simulink subsystem "BatteryHighGroupedRefSub"  (R2022a)
settings: Solver=VariableStepAuto  StartTime=0.0  StopTime=10.0  RelTol=1e-3
undefined symbols (not defined in the file): batteryHV
libraries: fl_lib x8, nesl_utility x7, batteryModule_lib x1
settings Model: Creator=jjha  LastModifiedBy=jjha
settings SolverCC: AlgebraicLoopSolver=TrustRegion
settings DebuggingCC: UnconnectedInputMsg=warning  UnconnectedOutputMsg=warning  UnconnectedLineMsg=warning
settings RTWCC: DLArmComputeVersion=19.05

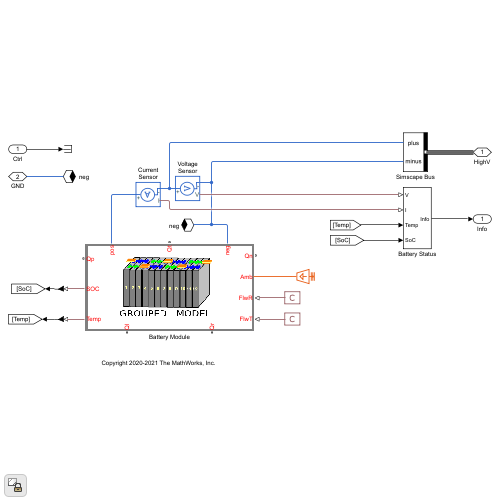
[thumbnail: Simulink's stored preview of the top-level diagram]
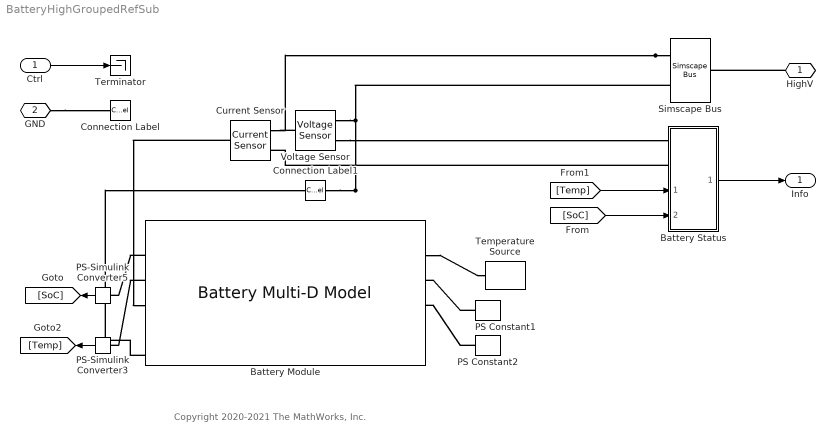
== system BatteryHighGroupedRefSub ==
  note: Copyright 2020-2021 The MathWorks, Inc.
  Ctrl : Inport
  Battery Module : batteryModule_lib/Battery Multi-D Model  modelComplexity=batteryModule.batteryAbstractionLevel.grouped  LUTpointsTemp=batteryHV.batteryTemp_LUT K  cellAH=batteryHV.batteryCapacity_LUT A*hr  LUTpointsSOC=batteryHV.batterySOC_LUT  V0_mat=batteryHV.batteryEm_LUT V  prm_dir=ee.enum.battery.prm_dir.noCurrentDirectionality  R0_mat=batteryHV.batteryR0_LUT Ohm  R0_dis_mat=[.03, .015, .002; .04, .017, .008; .039, .012, .006; .027, .013, .021] Ohm  R0_ch_mat=[.03, .015, .002; .04, .017, .008; .039, .012, .006; .027, .013, .021] Ohm  prm_leak=ee.enum.battery.prm_leak.disabled  Rleak_vec=[8000, 7000, 6000] Ohm  extrapolation_option=simscape.enum.extrapolation.nearest  prm_dyn=ee.enum.battery.prm_dyn.rc1  R1_mat=batteryHV.batteryR1_LUT Ohm  tau1_mat=batteryHV.batteryTau1_LUT s  R2_mat=[.014, .382, .407; .028, .006, .007; .014, .007, .006; .333, .956, .912] Ohm  tau2_mat=[1, 44, 5644; 11, 24, 506; 2, 14, 330; 3310, 13419, 30216] s  R3_mat=[.014, .382, .407; .028, .006, .007; .014, .007, .006; .333, .956, .912] Ohm  tau3_mat=[1, 44, 5644; 11, 24, 506; 2, 14, 330; 3310, 13419, 30216] s  R4_mat=[.014, .382, .407; .028, .006, .007; .014, .007, .006; .333, .956, .912] Ohm  tau4_mat=[1, 44, 5644; 11, 24, 506; 2, 14, 330; 3310, 13419, 30216] s  R5_mat=[.014, .382, .407; .028, .006, .007; .014, .007, .006; .333, .956, .912] Ohm  tau5_mat=[1, 44, 5644; 11, 24, 506; 2, 14, 330; 3310, 13419, 30216] s  prm_fade=ee.enum.battery.prm_fade.equations  N0=100  dV0=0  dR0=0  dAH=0  dRleak=0  dR1=0  dR2=0  dR3=0  dR4=0  dR5=0  N0vec=[100, 200, 300]  Tfadevec=[298.15, 323.15] K  dV0vec=[0, 0, 0]  dR0vec=[0, 0, 0]  dAHvec=[0, 0, 0]  dRleakvec=[0, 0, 0]  dR1vec=[0, 0, 0]  dR2vec=[0, 0, 0]  dR3vec=[0, 0, 0]  dR4vec=[0, 0, 0]  dR5vec=[0, 0, 0]  dV0mat=[0, 0; 0, 0; 0, 0]  dR0mat=[0, 0; 0, 0; 0, 0]  dAHmat=[0, 0; 0, 0; 0, 0]  dRleakmat=[0, 0; 0, 0; 0, 0]  dR1mat=[0, 0; 0, 0; 0, 0]  dR2mat=[0, 0; 0, 0; 0, 0]  dR3mat=[0, 0; 0, 0; 0, 0]  dR4mat=[0, 0; 0, 0; 0, 0]  dR5mat=[0, 0; 0, 0; 0, 0]  cellThermalMass=batteryHV.batteryCell_mass*batteryHV.batteryCell_cp J/K  cellThermalCond=batteryHV.batteryThermal_K1 W/(m*K)  cellThermalCond_inPlane=batteryHV.batteryThermal_K2 W/(m*K)  Ns=batteryHV.batteryNs  Np=batteryHV.batteryNp  cellTypeSelection=batteryModule.batteryTypeSelection.pouch  cellHeight=batteryHV.batteryCell_H m  cellWidth=batteryHV.batteryCell_W m  cellThickness=batteryHV.batteryCell_T m  cellDiameter=0.018 m  cellCylinLine=3  moduleExternalR=batteryHV.battery_extR Ohm  moduleCellBalancing=batteryModule.batteryCellBalancing.none  passiveShuntR=50 Ohm  passiveSWclosedR=0.01 Ohm  passiveSWopenCond=1e-8 1/Ohm  passiveSWthreshold=0.5  moduleCellVoltages=batteryModule.batteryCellVoltages.no  thermalManagement=batteryModule.batteryCoolingSystem.thermalPort  cellHeatTrCoeff=1 W/(m^2 * K)  thermal_moduleBottom=batteryModule.batteryThermalPortSelection.thermalLUT  htc_bottom=1 W/(m^2 * K)  moduleCooling_b=batteryHV.batteryCoolantHTC W/K  LUTpointsFlowrate_b=batteryHV.batteryCoolant_flow kg/s  LUTpointsTemp_b=batteryHV.batteryTemp_LUT K  thermal_moduleTop=batteryModule.batteryThermalPortSelection.thermalPortLumped  htc_top=batteryHV.batteryModuleTopHTC W/(m^2 * K)  moduleCooling_t=batteryHV.batteryCoolantHTC W/K  LUTpointsFlowrate_t=batteryHV.batteryCoolant_flow kg/s  LUTpointsTemp_t=batteryHV.batteryTemp_LUT K  thermal_moduleRight=batteryModule.batteryThermalPortSelection.thermalPortLumped  htc_right=1 W/(m^2 * K)  moduleCooling_r=zeros(3,6,batteryHV.batteryNs*batteryHV.batteryNp) W/K  LUTpointsFlowrate_r=[.01, .02, .03, .04, .05, .06] kg/s  LUTpointsTemp_r=[273.15, 298.15, 323.15] K  thermal_moduleLeft=batteryModule.batteryThermalPortSelection.thermalPortLumped  htc_left=1 W/(m^2 * K)  moduleCooling_l=zeros(3,6,batteryHV.batteryNs*batteryHV.batteryNp) W/K  LUTpointsFlowrate_l=[.01, .02, .03, .04, .05, .06] kg/s  LUTpointsTemp_l=[273.15, 298.15, 323.15] K  thermal_modulePos=batteryModule.batteryThermalPortSelection.thermalPortLumped  htc_pos=1 W/(m^2 * K)  moduleCooling_p=zeros(3,6,batteryHV.batteryNs*batteryHV.batteryNp) W/K  LUTpointsFlowrate_p=[.01, .02, .03, .04, .05, .06] kg/s  LUTpointsTemp_p=[273.15, 298.15, 323.15] K  thermal_moduleNeg=batteryModule.batteryThermalPortSelection.thermalPortLumped  htc_neg=1 W/(m^2 * K)  moduleCooling_n=zeros(3,6,batteryHV.batteryNs*batteryHV.batteryNp) W/K  LUTpointsFlowrate_n=[.01, .02, .03, .04, .05, .06] kg/s  LUTpointsTemp_n=[273.15, 298.15, 323.15] K  moduleExtHeat=batteryHV.batteryModuleExtHeat W  cellTemp=batteryHV.batteryModuleCellT_ini K  cellSOC=batteryHV.batteryModuleCellSOC_ini  moduleCellAHpercentVar=batteryHV.batteryModuleCellAhr_ini  moduleCellLeakPercentVar=ones(1, 10)  moduleCellR0PercentVar=batteryHV.batteryModuleCellR0_ini
      settings: InternalSimscapePortConfiguration="{\"Bottom\":[{\"id\":\"Ql\",\"label\":\"Ql\",\"type\":\"foundation.thermal.thermal\"},{\"id\":\"Qr\",\"label\":\"Qr\",\"type\":\"foundation.thermal.thermal\"}],\"Left\":[{\"id\":\"Qp\",\"label\":\"Qp\",\"type\":\"foundation.thermal.thermal\"},{\"id\":\"outputCellSOC\",\"label\":\"SOC\",\"type\":\"output\"},{\"id\":\"outputCellTemp\",\"label\":\"Temp\",\"type\":\"output\"}],\"Right\":[{\"id\":\"Qn\",\"label\":\"Qn\",\"type\":\"foundation.thermal.thermal\"},{\"id\":\"H\",\"label\":\"Amb\",\"type\":\"foundation.thermal.thermal\"},{\"id\":\"frac_b\",\"label\":\"FlwR\",\"type\":\"input\"},{\"id\":\"delT_b\",\"label\":\"FlwT\",\"type\":\"input\"}],\"Top\":[{\"id\":\"p\",\"label\":\"pos\",\"type\":\"foundation.electrical.electrical\"},{\"id\":\"Qt\",\"label\":\"Qt\",\"type\":\"foundation.thermal.thermal\"},{\"id\":\"n\",\"label\":\"neg\",\"type\":\"foundation.electrical.electrical\"}]}"
  Battery Status : Subsystem
      settings: PortSchema="{\"entries\":[{\"content\":{\"sides\":[{\"content\":{\"connectorIds\":[\"LConn1\",\"LConn2\",\"In1\",\"In2\"]},\"type\":\"ConnectorPlacement.EquallySpacedRectSide\",\"uuid\":\"240b64a7-8d8e-4535-9e7b-48cd07df38a6\"},{\"content\":{\"connectorIds\":[\"Out1\"],\"side\":\"RIGHT\"},\"type\":\"ConnectorPlacement.EquallySpacedRectSide\",\"uuid\":\"1719e6a6-4d63-4b0d-b06e-cf72ce82e787\"},{\"content\":{\"connectorIds\":[],\"side\":\"TOP\"},\"type\":\"ConnectorPlacement.EquallySpacedRectSide\",\"uuid\":\"7e887641-f2ac-443e-af1e-1937de5a1307\"},{\"content\":{\"connectorIds\":[],\"side\":\"BOTTOM\"},\"type\":\"ConnectorPlacement.EquallySpacedRectSide\",\"uuid\":\"5404d9ce-f296-45f3-ae79-f0f38b80df4c\"},{\"content\":{\"connectorIds\":[],\"side\":\"HIDDEN\"},\"type\":\"ConnectorPlacement.EquallySpacedRectSide\",\"uuid\":\"5562c952-4517-4b24-9dd4-ff12742a4401\"}]},\"type\":\"ConnectorPlacement.EquallySpacedConnector\",\"uuid\":\"fae3f649-0c67-4bb5-a707-519beddf154b\"}],\"packageUris\":[\"http://schema.mathworks.com/mf0/Connector/R2020b\"],\"version\":\"1.0\"}"
  Connection Label : ConnectionLabel  Label=neg
  Connection Label1 : ConnectionLabel  Label=neg
  Current Sensor : fl_lib/Electrical/Electrical Sensors/Current Sensor
      settings: SourceProductBaseCode=PW,SS,VE
  PS Constant1 : fl_lib/Physical Signals/Sources/PS Constant  constant=batteryHV.batteryCoolantFlwR
      settings: SourceProductBaseCode=PW,SS,VE
  PS Constant2 : fl_lib/Physical Signals/Sources/PS Constant  constant=batteryHV.batteryCoolantFlwT K
      settings: SourceProductBaseCode=PW,SS,VE
  PS-Simulink Converter3 : nesl_utility/PS-Simulink Converter  PhysicalDomain=network_engine_domain  SubClassName=ps_output  LeftPortType=input  RightPortType=output  PseudoPeriodic=off  Frequencies=[]  VectorFormat=1-D array  Unit=K  AffineConversion=off
      settings: SourceProductBaseCode=SS,PW,VE
  PS-Simulink Converter5 : nesl_utility/PS-Simulink Converter  PhysicalDomain=network_engine_domain  SubClassName=ps_output  LeftPortType=input  RightPortType=output  PseudoPeriodic=off  Frequencies=[]  VectorFormat=1-D array  Unit=1  AffineConversion=off
      settings: SourceProductBaseCode=SS,PW,VE
  Simscape Bus : SimscapeBus  HierarchyStrings=plus;minus
  Temperature Source : fl_lib/Thermal/Thermal Sources/Temperature Source  temperature=293.15 K
      settings: SourceProductBaseCode=PW,SS,VE
  Terminator : Terminator
  Voltage Sensor : fl_lib/Electrical/Electrical Sensors/Voltage Sensor
      settings: SourceProductBaseCode=PW,SS,VE
  HighV : PMIOPort  Side=Right
  GND : PMIOPort  Port=2  Side=Left
  Info : Outport
  wires:
  Battery Status/1(Info) -> Info/1
  Ctrl/1 -> Terminator/1
  PS-Simulink Converter5/1 -> [SoC]
  PS-Simulink Converter3/1 -> [Temp]
  [SoC] -> Battery Status/2(SoC)
  [Temp] -> Battery Status/1(Temp)
  connections:
  Simscape Bus/LConn2 -- Connection Label1/LConn1 -- Battery Module/LConn6 -- Voltage Sensor/RConn2
  Simscape Bus/LConn1 -- Voltage Sensor/LConn1 -- Current Sensor/RConn2
  Current Sensor/LConn1 -- Battery Module/LConn4
  HighV/RConn1 -- Simscape Bus/RConn1
  Voltage Sensor/RConn1 -- Battery Status/LConn1
  Battery Status/LConn2 -- Current Sensor/RConn1
  Battery Module/RConn2 -- Temperature Source/LConn1
  Battery Module/LConn3 -- PS-Simulink Converter3/LConn1
  GND/RConn1 -- Connection Label/LConn1
  Battery Module/LConn2 -- PS-Simulink Converter5/LConn1
  PS Constant1/RConn1 -- Battery Module/RConn3
  PS Constant2/RConn1 -- Battery Module/RConn4

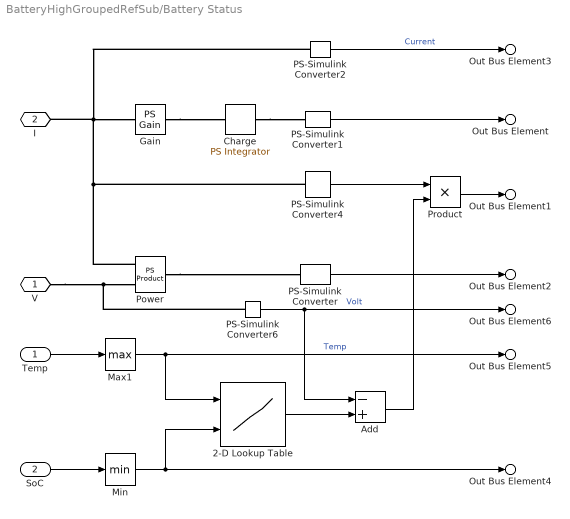
== system BatteryHighGroupedRefSub/Battery Status ==
  Temp : Inport
  SoC : Inport  Port=2
  2-D Lookup Table : Lookup_n-D  BreakpointsForDimension1=batteryHV.batterySOC_LUT  BreakpointsForDimension2=batteryHV.batteryTemp_LUT  Table=batteryHV.batteryEm_LUT  InternalRulePriority=Speed  RndMeth=Simplest
      settings: InputPortMap=u0,u1
  Add : Sum  Inputs=-+
  Charge : fl_lib/Physical Signals/Linear Operators/PS Integrator  reset_method=foundation.enum.IntegratorResetSpec.None  initial_condition_spec=foundation.enum.IntegratorICSpec.Internal  x0=batteryHV.batteryPackAhr_ini A*hr
      settings: SourceProductBaseCode=PW,SS,VE
  Gain : fl_lib/Physical Signals/Functions/PS Gain  gain=-1
      settings: AttributesFormatString=%<gain>  SourceProductBaseCode=PW,SS,VE
  Max1 : MinMax  Function=max
  Min : MinMax
  PS-Simulink Converter : nesl_utility/PS-Simulink Converter  PhysicalDomain=network_engine_domain  SubClassName=ps_output  LeftPortType=input  RightPortType=output  PseudoPeriodic=off  Frequencies=[]  VectorFormat=1-D array  Unit=kW  AffineConversion=off
      settings: SourceProductBaseCode=SS,PW,VE
  PS-Simulink Converter1 : nesl_utility/PS-Simulink Converter  PhysicalDomain=network_engine_domain  SubClassName=ps_output  LeftPortType=input  RightPortType=output  PseudoPeriodic=off  Frequencies=[]  VectorFormat=1-D array  Unit=A*hr  AffineConversion=off
      settings: SourceProductBaseCode=SS,PW,VE
  PS-Simulink Converter2 : nesl_utility/PS-Simulink Converter  PhysicalDomain=network_engine_domain  SubClassName=ps_output  LeftPortType=input  RightPortType=output  PseudoPeriodic=off  Frequencies=[]  VectorFormat=1-D array  Unit=A  AffineConversion=off
      settings: SourceProductBaseCode=SS,PW,VE
  PS-Simulink Converter4 : nesl_utility/PS-Simulink Converter  PhysicalDomain=network_engine_domain  SubClassName=ps_output  LeftPortType=input  RightPortType=output  PseudoPeriodic=off  Frequencies=[]  VectorFormat=1-D array  Unit=A  AffineConversion=off
      settings: SourceProductBaseCode=SS,PW,VE
  PS-Simulink Converter6 : nesl_utility/PS-Simulink Converter  PhysicalDomain=network_engine_domain  SubClassName=ps_output  LeftPortType=input  RightPortType=output  PseudoPeriodic=off  Frequencies=[]  VectorFormat=1-D array  Unit=V  AffineConversion=off
      settings: SourceProductBaseCode=SS,PW,VE
  Power : fl_lib/Physical Signals/Functions/PS Product
      settings: SourceProductBaseCode=PW,SS,VE
  Product : Product
  V : PMIOPort  Side=Left
  I : PMIOPort  Port=2  Side=Left
  Out Bus Element : Outport  PortName=Info  Element=Charge
      settings: AttributesFormatString=%<Unit>
  Out Bus Element1 : Outport  PortName=Info  Element=PowerLoss
      settings: AttributesFormatString=%<Unit>
  Out Bus Element2 : Outport  PortName=Info  Element=Power
      settings: AttributesFormatString=%<Unit>
  Out Bus Element3 : Outport  PortName=Info  Element=Current
      settings: AttributesFormatString=%<Unit>
  Out Bus Element4 : Outport  PortName=Info  Element=BatSoC
      settings: AttributesFormatString=%<Unit>
  Out Bus Element5 : Outport  PortName=Info  Element=BatTemp
      settings: AttributesFormatString=%<Unit>
  Out Bus Element6 : Outport  PortName=Info  Element=Volt
      settings: AttributesFormatString=%<Unit>
  wires:
  Max1/1 -> 2-D Lookup Table/1, Out Bus Element5/1  "Temp"
  Min/1 -> 2-D Lookup Table/2, Out Bus Element4/1
  Add/1 -> Product/2
  PS-Simulink Converter6/1 -> Add/1, Out Bus Element6/1  "Volt"
  2-D Lookup Table/1 -> Add/2
  PS-Simulink Converter4/1 -> Product/1
  Product/1 -> Out Bus Element1/1
  PS-Simulink Converter1/1 -> Out Bus Element/1
  PS-Simulink Converter/1 -> Out Bus Element2/1
  PS-Simulink Converter2/1 -> Out Bus Element3/1  "Current"
  Temp/1 -> Max1/1
  SoC/1 -> Min/1
  connections:
  PS-Simulink Converter4/LConn1 -- I/RConn1 -- PS-Simulink Converter2/LConn1 -- Gain/LConn1 -- Power/LConn2
  V/RConn1 -- PS-Simulink Converter6/LConn1 -- Power/LConn1
  Power/RConn1 -- PS-Simulink Converter/LConn1
  Charge/RConn1 -- PS-Simulink Converter1/LConn1
  Gain/RConn1 -- Charge/LConn1
